simulink model "absmdl_TypeB_CS9"  (Simulink 7.6)
settings: Solver=ode45  SolverMode=SingleTasking  StartTime=0  StopTime=8  FixedStep=0.002  RelTol=1e-3  AbsTol=1e-6
libraries: Solver_SF x1
settings Model: Creator=pmather  LastModifiedBy=hkawanishi  ExtModeTrigMode=oneshot  ExtModeArmWhenConnect=off
settings DataIOCC: LimitDataPoints=off
settings OptimizationCC: BlockReduction=off  BooleanDataType=off  InitFltsAndDblsToZero=on
settings DebuggingCC: SaveWithParameterizedLinksMsg=none  SignalResolutionControl=TryResolveAllWithWarning  SolverPrmCheckMsg=none  MultiTaskDSMMsg=warning  MultiTaskCondExecSysMsg=none  StrictBusMsg=None
settings HardwareCC: TargetUnknown=on
settings RTWCC: TemplateMakefile=grt_vc.tmf  IncludeERTFirstTime=on

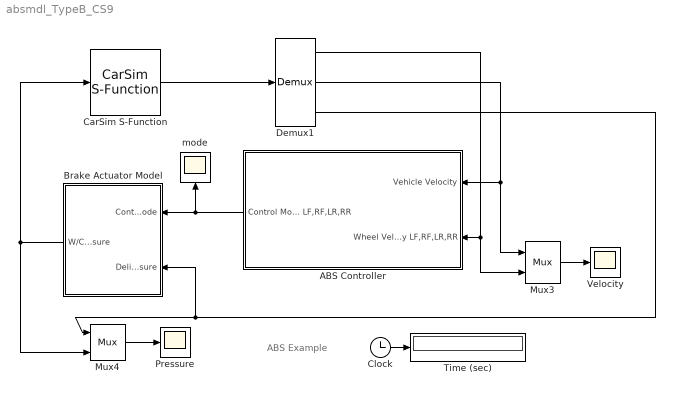
== system absmdl_TypeB_CS9 ==
  note: ABS Example
  ABS Controller : Subsystem
  Brake Actuator Model : Subsystem
  CarSim S-Function : Solver_SF/CarSim S-Function  Priority=1  SIMFILE=simfile.sim
  Clock : Clock
      settings: Decimation=10
  Demux1 : Demux  Outputs=[4 1 4]
  Mux3 : Mux  Inputs=2
  Mux4 : Mux  Inputs=2
  Pressure : Scope
      settings: TickLabels=on  YMin=0  YMax=20  DataFormat=Array  SampleTime=100
  Time (sec) : Display
      settings: Format=bank  Decimation=100
  Velocity : Scope
      settings: TickLabels=on  YMin=-10  YMax=100  DataFormat=Array  SampleTime=100
  mode : Scope
      settings: TickLabels=on  YMin=-1  YMax=1  DataFormat=Array  SampleTime=100
  wires:
  Mux4/1 -> Pressure/1
  CarSim S-Function/1 -> Demux1/1
  Demux1/2 -> Mux3/1, ABS Controller/1(Vehicle Velocity)
  Demux1/1 -> Mux3/2, ABS Controller/2(Wheel Velocity LF,RF,LR,RR)
  Clock/1 -> Time (sec)/1
  ABS Controller/1(Control Mode LF,RF,LR,RR) -> Brake Actuator Model/1(Control Mode), mode/1
  Brake Actuator Model/1(W/C Pressure) -> Mux4/2, CarSim S-Function/1
  Mux3/1 -> Velocity/1
  Demux1/3 -> Mux4/1, Brake Actuator Model/2(Delivery Pressure)

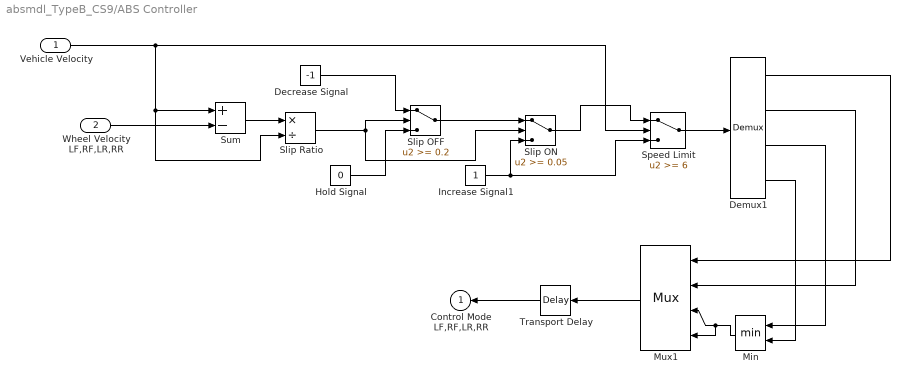
== system absmdl_TypeB_CS9/ABS Controller ==
  Vehicle Velocity : Inport
  Wheel Velocity LF,RF,LR,RR : Inport  Port=2
  Decrease Signal : Constant  Value=-1
  Demux1 : Demux
  Hold Signal : Constant  Value=0
  Increase Signal1 : Constant
  Min : MinMax  Inputs=2  SaturateOnIntegerOverflow=on  InputSameDT=on
  Mux1 : Mux
  Slip OFF : Switch  Threshold=0.2  SaturateOnIntegerOverflow=on  InputSameDT=on
  Slip ON : Switch  Threshold=0.05  SaturateOnIntegerOverflow=on  InputSameDT=on
  Slip Ratio : Product  Inputs=*/  SaturateOnIntegerOverflow=on  RndMeth=Zero  InputSameDT=on  OutDataTypeStr=Inherit: Same as first input
  Speed Limit : Switch  Threshold=6  SaturateOnIntegerOverflow=on  InputSameDT=on
  Sum : Sum  Inputs=+-  SaturateOnIntegerOverflow=on  InputSameDT=on  OutDataTypeStr=Inherit: Same as first input
  Transport Delay : TransportDelay  DelayTime=0.005
  Control Mode LF,RF,LR,RR : Outport  InitialOutput=0
  wires:
  Decrease Signal/1 -> Slip OFF/1
  Sum/1 -> Slip Ratio/1
  Wheel Velocity LF,RF,LR,RR/1 -> Sum/2
  Slip OFF/1 -> Slip ON/1
  Vehicle Velocity/1 -> Sum/1, Slip Ratio/2, Speed Limit/2
  Slip ON/1 -> Speed Limit/1
  Increase Signal1/1 -> Slip ON/3, Speed Limit/3
  Slip Ratio/1 -> Slip OFF/2, Slip ON/2
  Hold Signal/1 -> Slip OFF/3
  Transport Delay/1 -> Control Mode LF,RF,LR,RR/1
  Speed Limit/1 -> Demux1/1
  Min/1 -> Mux1/3, Mux1/4
  Demux1/2 -> Mux1/2
  Demux1/1 -> Mux1/1
  Mux1/1 -> Transport Delay/1
  Demux1/4 -> Min/2
  Demux1/3 -> Min/1

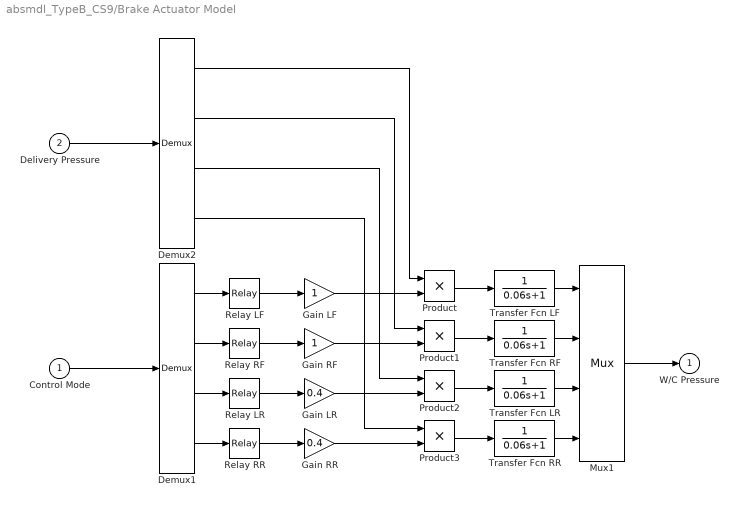
== system absmdl_TypeB_CS9/Brake Actuator Model ==
  Control Mode : Inport
  Delivery Pressure : Inport  Port=2
  Demux1 : Demux
  Demux2 : Demux
  Gain LF : Gain  SaturateOnIntegerOverflow=on  OutDataTypeStr=Inherit: Same as input  ParamDataTypeStr=Inherit: Same as input
  Gain LR : Gain  Gain=0.4  SaturateOnIntegerOverflow=on  OutDataTypeStr=Inherit: Same as input  ParamDataTypeStr=Inherit: Same as input
  Gain RF : Gain  SaturateOnIntegerOverflow=on  OutDataTypeStr=Inherit: Same as input  ParamDataTypeStr=Inherit: Same as input
  Gain RR : Gain  Gain=0.4  SaturateOnIntegerOverflow=on  OutDataTypeStr=Inherit: Same as input  ParamDataTypeStr=Inherit: Same as input
  Mux1 : Mux
  Product{,1..3} (4 alike) : Product  SaturateOnIntegerOverflow=on  RndMeth=Zero  InputSameDT=on  OutDataTypeStr=Inherit: Same as first input
  Relay LF : Relay  OnSwitchValue=0.5  OffSwitchValue=-0.5
  Relay LR : Relay  OnSwitchValue=0.5  OffSwitchValue=-0.5
  Relay RF : Relay  OnSwitchValue=0.5  OffSwitchValue=-0.5
  Relay RR : Relay  OnSwitchValue=0.5  OffSwitchValue=-0.5
  Transfer Fcn LF : TransferFcn  Denominator=[0.06 1]
  Transfer Fcn LR : TransferFcn  Denominator=[0.06 1]
  Transfer Fcn RF : TransferFcn  Denominator=[0.06 1]
  Transfer Fcn RR : TransferFcn  Denominator=[0.06 1]
  W/C Pressure : Outport  InitialOutput=0
  wires:
  Mux1/1 -> W/C Pressure/1
  Control Mode/1 -> Demux1/1
  Demux1/1 -> Relay LF/1
  Demux1/2 -> Relay RF/1
  Demux1/3 -> Relay LR/1
  Demux1/4 -> Relay RR/1
  Relay LF/1 -> Gain LF/1
  Relay RF/1 -> Gain RF/1
  Relay LR/1 -> Gain LR/1
  Relay RR/1 -> Gain RR/1
  Gain LF/1 -> Product/2
  Gain RF/1 -> Product1/2
  Gain LR/1 -> Product2/2
  Gain RR/1 -> Product3/2
  Product/1 -> Transfer Fcn LF/1
  Transfer Fcn LF/1 -> Mux1/1
  Product1/1 -> Transfer Fcn RF/1
  Product2/1 -> Transfer Fcn LR/1
  Product3/1 -> Transfer Fcn RR/1
  Transfer Fcn RF/1 -> Mux1/2
  Transfer Fcn LR/1 -> Mux1/3
  Transfer Fcn RR/1 -> Mux1/4
  Delivery Pressure/1 -> Demux2/1
  Demux2/1 -> Product/1
  Demux2/2 -> Product1/1
  Demux2/3 -> Product2/1
  Demux2/4 -> Product3/1
